simulink model "q3"  (R2020b)
settings: Solver=FixedStepAuto  StartTime=0.0  StopTime=10.0  RelTol=1e-3
settings Model: Creator=AVM  LastModifiedBy=AVM

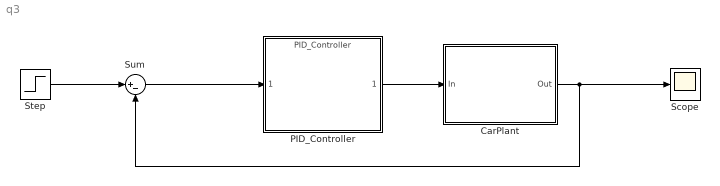
== system q3 ==
  CarPlant : Subsystem
  PID_Controller : ModelReference  ModelNameDialog=PID_Controller  UsingDefaultArgumentValue=0,0,0  SimulationMode=Normal  ModelReferenceVersion=1.10  Kd=346  Ki=76  Kp=1000  SimulationMode=Normal
  Scope : Scope
  Step : Step  After=10  SampleTime=0
  Sum : Sum  Inputs=|+-
  wires:
  CarPlant/1(Out) -> Scope/1, Sum/2
  Step/1 -> Sum/1
  Sum/1 -> PID_Controller/1
  PID_Controller/1 -> CarPlant/1(In)

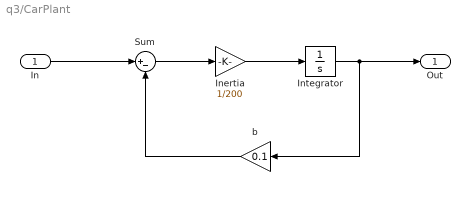
== system q3/CarPlant ==
  In : Inport
  Inertia : Gain  Gain=1/200
  Integrator : Integrator
  Sum : Sum  Inputs=|+-
  b : Gain  Gain=0.1
  Out : Outport
  wires:
  Inertia/1 -> Integrator/1
  Integrator/1 -> Out/1, b/1
  Sum/1 -> Inertia/1
  b/1 -> Sum/2
  In/1 -> Sum/1
